simulink model "modelsaw"  (R2019a)
settings: Solver=FixedStepAuto  StartTime=0.0  StopTime=0.1  FixedStep=1e-5  RelTol=1e-3
libraries: simulink x3
settings Model: Creator=Sherlock Holmes  LastModifiedBy=Sherlock Holmes

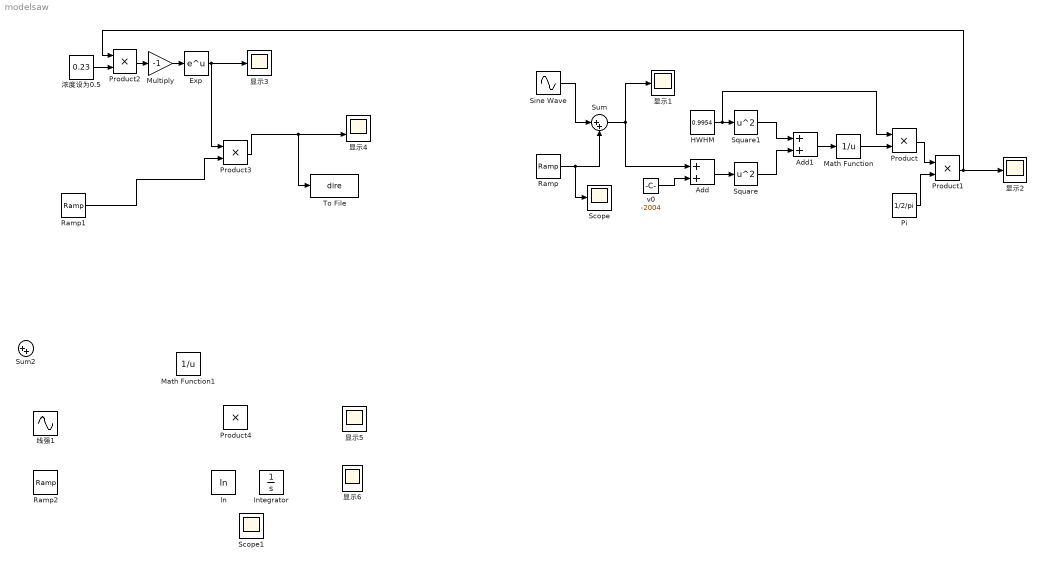
== system modelsaw ==
  Add : Sum
  Add1 : Sum
  Exp : Math  SaturateOnIntegerOverflow=on
  HWHM : Constant  Value=0.9954  OutDataTypeStr=Inherit: Inherit via back propagation
  Integrator : Integrator
  Math Function : Math  Operator=reciprocal  RndMeth=Zero  SaturateOnIntegerOverflow=on
  Math Function1 : Math  Operator=reciprocal  RndMeth=Zero  SaturateOnIntegerOverflow=on
  Multiply : Gain  Gain=-1
  Pi : Constant  Value=1/2/pi  OutDataTypeStr=Inherit: Inherit via back propagation
  Product{,1..4} (5 alike) : Product
  Ramp : simulink/Sources/Ramp  slope=80  start=0  InitialOutput=2000
  Ramp1 : simulink/Sources/Ramp  slope=21  start=0  InitialOutput=2
  Ramp2 : simulink/Sources/Ramp  slope=21  start=0  InitialOutput=2
  Scope : Scope
  Scope1 : Scope
  Sine Wave : Sin  Amplitude=0.1  Frequency=5000  SampleTime=0
  Square : Math  Operator=square  SaturateOnIntegerOverflow=on
  Square1 : Math  Operator=square  SaturateOnIntegerOverflow=on
  Sum : Sum  Inputs=|++
  Sum2 : Sum  Inputs=|++
  To File : ToFile  Filename=dire  MatrixName=direData  SaveFormat=Timeseries
  ln : Math  Operator=log  SaturateOnIntegerOverflow=on
  v0 : Constant  Value=-2004  OutDataTypeStr=Inherit: Inherit via back propagation
  显示{1..3,5..6} (5 alike) : Scope
  显示4 : Scope  NumInputPorts=2
  浓度设为0.5 : Constant  Value=0.23  OutDataTypeStr=Inherit: Inherit via back propagation
  线强1 : Sin  Amplitude=0.1  Frequency=5000  SampleTime=0
  wires:
  Sine Wave/1 -> Sum/1
  Ramp/1 -> Scope/1, Sum/2
  Sum/1 -> 显示1/1, Add/1
  v0/1 -> Add/2
  HWHM/1 -> Product/1, Square1/1
  Add/1 -> Square/1
  Square1/1 -> Add1/1
  Square/1 -> Add1/2
  Add1/1 -> Math Function/1
  Math Function/1 -> Product/2
  Product/1 -> Product1/1
  Pi/1 -> Product1/2
  Product1/1 -> Product2/1, 显示2/1
  浓度设为0.5/1 -> Product2/2
  Exp/1 -> Product3/1, 显示3/1
  Ramp1/1 -> Product3/2
  Product3/1 -> To File/1, 显示4/2
  Product2/1 -> Multiply/1
  Multiply/1 -> Exp/1
